simulink model "chap8_9sim"  (Simulink 7.7)
settings: Solver=ode45  StartTime=0.0  StopTime=10  RelTol=1e-3
settings Model: Creator=ljk  LastModifiedBy=ljk  ExtModeTrigMode=oneshot  ExtModeArmWhenConnect=off
settings DataIOCC: LimitDataPoints=off
settings OptimizationCC: BlockReduction=off  BooleanDataType=off
settings DebuggingCC: SaveWithParameterizedLinksMsg=none  SignalResolutionControl=TryResolveAllWithWarning  SolverPrmCheckMsg=none  MultiTaskDSMMsg=warning  MultiTaskCondExecSysMsg=none  StrictBusMsg=None
settings HardwareCC: TargetUnknown=on
settings RTWCC: IncludeERTFirstTime=on

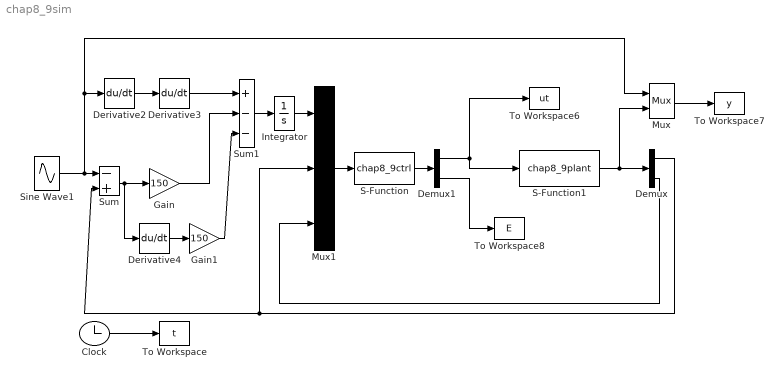
== system chap8_9sim ==
  Clock : Clock
  Demux : Demux  Outputs=2
  Demux1 : Demux  Outputs=2
  Derivative2 : Derivative
  Derivative3 : Derivative
  Derivative4 : Derivative
  Gain : Gain  Gain=150  SaturateOnIntegerOverflow=on  OutDataTypeStr=Inherit: Same as input  ParamDataTypeStr=Inherit: Same as input
  Gain1 : Gain  Gain=150  SaturateOnIntegerOverflow=on  OutDataTypeStr=Inherit: Same as input  ParamDataTypeStr=Inherit: Same as input
  Integrator : Integrator
  Mux : Mux  Inputs=2
  Mux1 : Mux  Inputs=3
  S-Function : S-Function  FunctionName=chap8_9ctrl  EnableBusSupport=off
  S-Function1 : S-Function  FunctionName=chap8_9plant  EnableBusSupport=off
  Sine Wave1 : Sin  Amplitude=0.2  Frequency=pi  Phase=pi/2  SampleTime=0
  Sum : Sum  Inputs=-+  SaturateOnIntegerOverflow=on  InputSameDT=on  OutDataTypeStr=Inherit: Same as first input
  Sum1 : Sum  Inputs=+--  SaturateOnIntegerOverflow=on  InputSameDT=on  OutDataTypeStr=Inherit: Same as first input
  To Workspace : ToWorkspace  VariableName=t  SampleTime=-1  SaveFormat=Array
  To Workspace6 : ToWorkspace  VariableName=ut  SampleTime=-1  SaveFormat=Array
  To Workspace7 : ToWorkspace  VariableName=y  SampleTime=-1  SaveFormat=Array
  To Workspace8 : ToWorkspace  VariableName=E  SampleTime=-1  SaveFormat=Array
  wires:
  Derivative4/1 -> Gain1/1
  Sine Wave1/1 -> Sum/1, Derivative2/1, Mux/1
  Sum/1 -> Gain/1, Derivative4/1
  Derivative2/1 -> Derivative3/1
  Derivative3/1 -> Sum1/1
  Gain/1 -> Sum1/2
  Gain1/1 -> Sum1/3
  Clock/1 -> To Workspace/1
  Mux1/1 -> S-Function/1
  Integrator/1 -> Mux1/1
  Sum1/1 -> Integrator/1
  S-Function/1 -> Demux1/1
  Mux/1 -> To Workspace7/1
  Demux/1 -> Sum/2, Mux1/2
  Demux/2 -> Mux1/3
  Demux1/1 -> To Workspace6/1, S-Function1/1
  Demux1/2 -> To Workspace8/1
  S-Function1/1 -> Demux/1, Mux/2
